simulink model "lab8"  (R2023b)
settings: Solver=ode45  StartTime=0.0  StopTime=15.0  MaxStep=0.02  MinStep=0.01  RelTol=1e-3
settings Model: Creator=insomnia  LastModifiedBy=insomnia
settings SolverCC: InitialStep=0.01

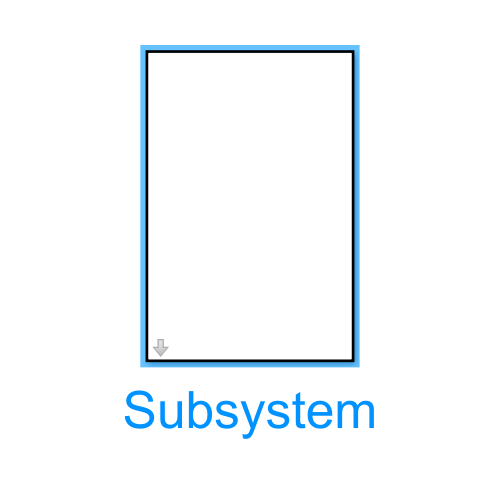
[thumbnail: Simulink's stored preview of the top-level diagram]
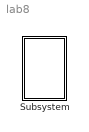
== system lab8 ==
  Subsystem : Subsystem  mask{g=9.81, k=1, m=2, l=4, xi=[-1 1 1], yi=[1 1 -1], di=[0.1 0.1 0.1], ai=[1 -1 1.5], x10=0, y10=0}
      mask prompts: g "przyspieszenie ziemskie"; k "wsp. tlumienia"; m "masa wahadla"; l "dlugosc linki wahadla"; xi "polozenie x magnesow"; yi "polozenie y magnesow"; di "odleglosc magnesow od plaszczyzny XY"; ai "sila z jaka magnesy oddzialuja na wahadlo"; x10 "x'(0)"; y10 "y'(0)"

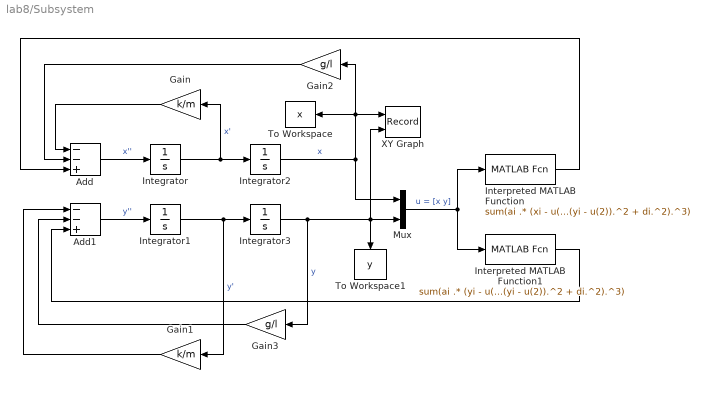
== system lab8/Subsystem ==
  Add : Sum  Inputs=--+
  Add1 : Sum  Inputs=--+
  Gain : Gain  Gain=k/m
  Gain1 : Gain  Gain=k/m
  Gain2 : Gain  Gain=g/l
  Gain3 : Gain  Gain=g/l
  Integrator : Integrator  InitialCondition=x10
  Integrator1 : Integrator  InitialCondition=y10
  Integrator2 : Integrator  InitialCondition=-1
  Integrator3 : Integrator  InitialCondition=-1
  Interpreted MATLAB Function : MATLABFcn  MATLABFcn=sum(ai .* (xi - u(1)) ./ sqrt((xi - u(1)).^2 + (yi - u(2)).^2 + di.^2).^3)
  Interpreted MATLAB Function1 : MATLABFcn  MATLABFcn=sum(ai .* (yi - u(2)) ./ sqrt((xi - u(1)).^2 + (yi - u(2)).^2 + di.^2).^3)
  Mux : Mux  Inputs=2
  To Workspace : ToWorkspace  VariableName=x  SampleTime=-1
  To Workspace1 : ToWorkspace  VariableName=y  SampleTime=-1
  XY Graph : Record  FileSettingsInternal="{\"entries\":[{\"content\":{\"excelSettings\":{\"content\":{},\"type\":\"Streamout.ExcelSettings\"}},\"type\":\"Streamout.FileSettingStorage\",\"uuid\":\"\"}],\"packageUris\":[\"http:\\/\\/schema.mathworks.com\\/mf0\\/streamout_blocks\\/R2020a\"],\"version\":\"1.0\"}"  Layout=[1 1]  SignalsInternal="{\"entries\":[{\"content\":{\"signals\":[{\"content\":{\"blockPath\":[],\"dimensions\":[1],\"domain\":\"\",\"lineColor\":\"#a2142f\",\"plots\":[ 1 ],\"port\":1,\"sid\":[\"\"],\"signalID\":1,\"signalName\":\"x\"},\"type\":\"RecordBlkView.Signal\",\"uuid\":\"\"},{\"content\":{\"blockPath\":[],\"dimensions\":[1],\"domain\":\"\",\"lineColor\":\"#139fff\",\"plots\":[ 1 ],\"port\":2,\"sid\":[\"\"],\"signalID\":2,\"signalName\":\"y\"},\"type\":\"RecordBlkView.Signal\",\"uuid\":\"\"}]},\"type\":\"RecordBlkView.InputSignals\",\"uuid\":\"\"}],\"packageUris\":[\"http:\\/\\/schema.mathworks.com\\/mf0\\/streamout_blocks\\/R2020a\"],\"version\":\"1.0\"}"  VisualizationBindings="{\"xyplotplugin\":{\"info\":[{\"series\":[{\"bindingParametersList\":[{\"parameter\":\"X-Axis\",\"signalID\":1,\"signalName\":\"x\"},{\"parameter\":\"Y-Axis\",\"signalID\":2,\"signalName\":\"y\"}],\"seriesID\":0}],\"subplotID\":1}]}}"  CompatibilityTag=XY
  wires:
  Integrator1/1 -> Gain1/1, Integrator3/1  "y'"
  Integrator2/1 -> To Workspace/1, XY Graph/1, Gain2/1, Mux/1  "x"
  Integrator/1 -> Gain/1, Integrator2/1  "x'"
  Add/1 -> Integrator/1  "x''"
  Mux/1 -> Interpreted MATLAB Function1/1, Interpreted MATLAB Function/1  "u = [x y]"
  Integrator3/1 -> Gain3/1, To Workspace1/1, XY Graph/2, Mux/2  "y"
  Gain2/1 -> Add/2
  Gain1/1 -> Add1/1
  Interpreted MATLAB Function/1 -> Add/3
  Gain/1 -> Add/1
  Interpreted MATLAB Function1/1 -> Add1/3
  Add1/1 -> Integrator1/1  "y''"
  Gain3/1 -> Add1/2
